simulink model "network_components"  (R2025b)
settings: Solver=VariableStepAuto  StartTime=0.0  StopTime=10.0  RelTol=1e-3
undefined symbols (not defined in the file or in its folder): Bpu, lineParam, Rpu
libraries: ee_lib x8, fl_lib x8, nesl_utility x4, ee_lib_for_power_systems x2
settings Model: Creator=gdudgeon  LastModifiedBy=gdudgeon

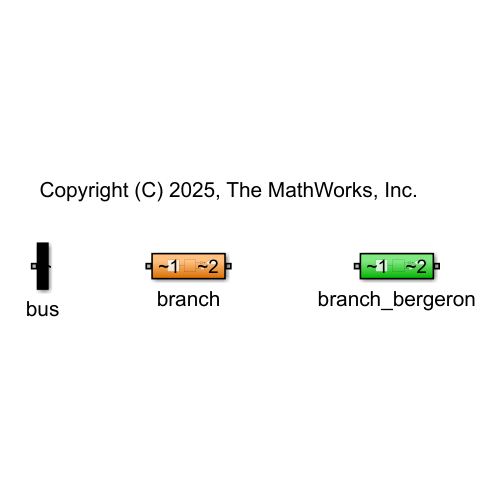
[thumbnail: Simulink's stored preview of the top-level diagram]
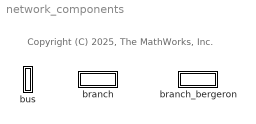
== system network_components ==
  note: Copyright (C) 2025, The MathWorks, Inc.
  branch : Subsystem
  branch_bergeron : Subsystem
  bus : Subsystem

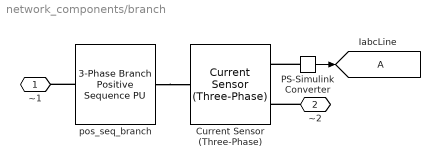
== system network_components/branch ==
  Current Sensor (Three-Phase) : ee_lib/Sensors & Transducers/Current Sensor (Three-Phase)
  IabcLine : Goto  TagVisibility=global
  PS-Simulink Converter : nesl_utility/PS-Simulink Converter  PhysicalDomain=network_engine_domain  SubClassName=ps_output  LeftPortType=input  RightPortType=output  PseudoPeriodic=off  Frequencies=[]  VectorFormat=inherit  Unit=inherit  AffineConversion=off
  pos_seq_branch : ee_lib_for_power_systems/Network Components/3-Phase Branch Positive Sequence PU  Pnom_Fnom=[5e6 60]  Tx=off  Vnom1=5e3  Vnom2=2e3  R=Rpu  X=Xpu  B=Bpu  run_time=on
      settings: SourceProductName=Support Library for Power Systems
  ~1 : PMIOPort  Side=Left
  ~2 : PMIOPort  Port=2  Side=Right
  wires:
  PS-Simulink Converter/1 -> IabcLine/1
  connections:
  PS-Simulink Converter/LConn1 -- Current Sensor (Three-Phase)/RConn1
  ~2/RConn1 -- Current Sensor (Three-Phase)/RConn2
  pos_seq_branch/RConn1 -- Current Sensor (Three-Phase)/LConn1
  pos_seq_branch/LConn1 -- ~1/RConn1

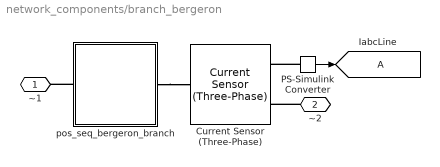
== system network_components/branch_bergeron ==
  Current Sensor (Three-Phase) : ee_lib/Sensors & Transducers/Current Sensor (Three-Phase)
  IabcLine : Goto  TagVisibility=global
  PS-Simulink Converter : nesl_utility/PS-Simulink Converter  PhysicalDomain=network_engine_domain  SubClassName=ps_output  LeftPortType=input  RightPortType=output  PseudoPeriodic=off  Frequencies=[]  VectorFormat=inherit  Unit=inherit  AffineConversion=off
  pos_seq_bergeron_branch : Subsystem  mask{Pnom_Fnom=[5e6 60], Tx=off, Vnom1=5e3, Vnom2=2e3, R=0.1, X=0.01, B=1e-9}
      mask prompts: Pnom_Fnom "Nominal values [Pnom(VA) Fnom(Hz)]"; Tx "Include Ideal Transformer"; Vnom1 "Port 1 Nominal Voltage (Vrms)"; Vnom2 "Nominal Voltage (Vrms)"; R "Series Resistance R (pu)"; X "Series Reactance X (pu)"; B "Shunt Line Charging Susceptance B (pu)"
      mask init:
      | maskObj = Simulink.Mask.get(gcbh);
      | workspaceObj = maskObj.getWorkspace();
      | 
      | Pnom_Vnom = workspaceObj.get('Pnom_Fnom');
      | Vnom1 = workspaceObj.get('Vnom1');
      | Vnom2 = workspaceObj.get('Vnom2');
      | 
      | R = workspaceObj.get('R');
      | X = workspaceObj.get('X');
      | B = workspaceObj.get('B');
      | 
      | R1 = R*Vnom2^2/Pnom_Fnom(1);
      | R0 = R1;
      | 
      | L1 = X*Vnom2^2/Pnom_Fnom(1)/(2*pi*Pnom_Fnom(2));
      | L0 = L1;
      | 
      | C1 = B/(Vnom2^2/Pnom_Fnom(1))/(2*pi*Pnom_Fnom(2));
      | C0 = C1;
      mask Callback Tx:
      | Tx = get_param(gcb,'Tx');
      | 
      | path_Tx  = [gcb,'/Tx'];
      | 
      | mp  ={
      |     'Nominal values [Pnom(VA) Fnom(Hz)]'
      |     'Include Ideal Transformer'
      |     'Port 1 Nominal Voltage (Vrms)'
      |     'Nominal Voltage (Vrms)'
      |     'Series Resistance R (pu)'
      |     'Series Reactance X (pu)'
      |     'Shunt Line Charging Susceptance B (pu)'
      |     };
      | 
      | set_param(gcb,'MaskPrompts',mp)
      | 
      | switch Tx
      | 
      |     case 'off'
      | 
      |         set_param(gcb,'MaskVisibilityString','on,on,off,on,on,on,on')
      |         set_param(path_Tx,'Commented','through')
      | 
      |     case 'on'
      | 
      |         set_param(gcb,'MaskVisibilityString','on,on,on,on,on,on,on')
      |         mp{4} = 'Port 2 Nominal Voltage (Vrms)';
      |         set_param(path_Tx,'Commented','off')
      | 
      | end
      | 
      | set_param(gcb,'MaskPrompts',mp)
      mask DialogControl DescGroupVar Prompt: 3-Phase Branch Positive Sequence PU
      mask DialogControl DescTextVar Prompt: This branch is parameterized from positive sequence data in R, X, B format. Where R is series resistance, X is series reactance and B is line charging susceptance. For series inductance X is positive. For series capacitance, X is negative. When included, the ideal transformer is connected at port 1, and the RLC per-unit values are referred to the voltage at port 2.
      mask DialogControl Container5 Prompt: Parameters
      mask Display: disp('Three-Phase\nBergeron\nPos-Seq (PU)')
  ~1 : PMIOPort  Side=Left
  ~2 : PMIOPort  Port=2  Side=Right
  wires:
  PS-Simulink Converter/1 -> IabcLine/1
  connections:
  pos_seq_bergeron_branch/LConn1 -- ~1/RConn1
  pos_seq_bergeron_branch/RConn1 -- Current Sensor (Three-Phase)/LConn1
  ~2/RConn1 -- Current Sensor (Three-Phase)/RConn2
  PS-Simulink Converter/LConn1 -- Current Sensor (Three-Phase)/RConn1

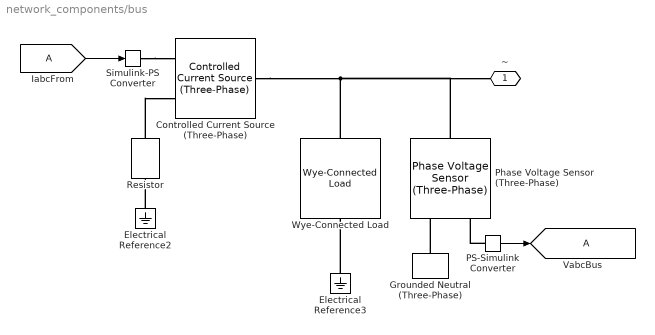
== system network_components/bus ==
  Controlled Current Source (Three-Phase) : ee_lib/Sources/Controlled Current Source (Three-Phase)  input_option=ee.enum.inputType.instantaneous  FRated=60 Hz
      settings: InternalSimscapePortConfiguration="{\"Bottom\":[],\"Left\":[{\"id\":\"S\",\"label\":\"S\",\"type\":\"input\"},{\"id\":\"n\",\"label\":\"n\",\"type\":\"foundation.electrical.electrical\"}],\"Right\":[{\"id\":\"N\",\"label\":\"~\",\"type\":\"foundation.electrical.three_phase\"}],\"Top\":[]}"
  Electrical Reference2 : fl_lib/Electrical/Electrical Elements/Electrical Reference
  Electrical Reference3 : fl_lib/Electrical/Electrical Elements/Electrical Reference
  Grounded Neutral (Three-Phase) : ee_lib/Connectors & References/Grounded Neutral (Three-Phase)
  IabcFrom : From
  PS-Simulink Converter : nesl_utility/PS-Simulink Converter  PhysicalDomain=network_engine_domain  SubClassName=ps_output  LeftPortType=input  RightPortType=output  PseudoPeriodic=off  Frequencies=[]  VectorFormat=inherit  Unit=inherit  AffineConversion=off
  Phase Voltage Sensor (Three-Phase) : ee_lib/Sensors & Transducers/Phase Voltage Sensor (Three-Phase)
  Resistor : fl_lib/Electrical/Electrical Elements/Resistor  R=lineParam.RgI Ohm  i_specify=on  i_priority=High  i=0 A  i_nominal_specify=off  i_nominal_value=1  i_nominal_unit=A  v_specify=on  v_priority=High  v=0 V  v_nominal_specify=off  v_nominal_value=1  v_nominal_unit=V
  Simulink-PS Converter : nesl_utility/Simulink-PS Converter  PhysicalDomain=network_engine_domain  SubClassName=ps_input  LeftPortType=input  RightPortType=output  PseudoPeriodic=off  Frequencies=[]  NoiseDistribution=none  NoiseParameters=[]  Unit=1  AffineConversion=off  FilteringAndDerivatives=zero  SimscapeFilterOrder=1  InputFilterTimeConstant=0.001  UdotUserProvided=0
  VabcBus : Goto  TagVisibility=global
  Wye-Connected Load : ee_lib/Passive/RLC Assemblies/Wye-Connected Load  port_option=ee.enum.threePhasePort.composite  parameterization=ee.enum.rlc.parameterization.ratedpower  component_structure=ee.enum.rlc.structure.R  component_structure_PQ=ee.enum.rlc.structure.ParallelRLC  R=1 Ohm  L=1e-3 H  C=1e-6 F  VRated=24e3 V  FRated=60 Hz  P=1e3 W  Qpos=1e2 A*V  Qneg=-1e2 A*V  R_parasitic=0 Ohm  G_parasitic=0 1/Ohm  R_parasitic_PQ=0 Ohm  G_parasitic_PQ=0 1/Ohm  Vmag0=0 V  Vang0=0 deg  Freq0=60 Hz  IL_specify=off  IL_priority=High  IL=[0, 0, 0] A  IL_nominal_specify=off  IL_nominal_value=1  IL_nominal_unit=A  VC_specify=off  VC_priority=High  VC=[0, 0, 0] V  VC_nominal_specify=off  VC_nominal_value=1  VC_nominal_unit=V
  ~ : PMIOPort  Side=Left
  wires:
  IabcFrom/1 -> Simulink-PS Converter/1
  PS-Simulink Converter/1 -> VabcBus/1
  connections:
  Wye-Connected Load/LConn1 -- Controlled Current Source (Three-Phase)/RConn1 -- Phase Voltage Sensor (Three-Phase)/LConn1 -- ~/RConn1
  Electrical Reference2/LConn1 -- Resistor/LConn1
  Electrical Reference3/LConn1 -- Wye-Connected Load/RConn1
  Simulink-PS Converter/RConn1 -- Controlled Current Source (Three-Phase)/LConn1
  PS-Simulink Converter/LConn1 -- Phase Voltage Sensor (Three-Phase)/RConn1
  Grounded Neutral (Three-Phase)/LConn1 -- Phase Voltage Sensor (Three-Phase)/RConn2
  Resistor/RConn1 -- Controlled Current Source (Three-Phase)/LConn2

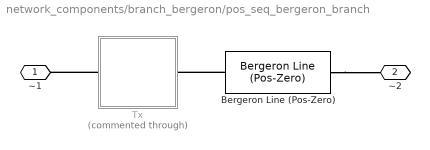
== system network_components/branch_bergeron/pos_seq_bergeron_branch ==
  Bergeron Line (Pos-Zero) : ee_lib_for_power_systems/Network Components/Bergeron Line (Pos-Zero)  length=1  R1_L1_C1=[R1 L1 C1]  R0_L0_C0=[R1 L1 C1]  Ts=5e-5
      settings: SourceProductName=Support Library for Power Systems
  Tx : Subsystem  Commented=through  mask{wr=Vnom1/Vnom2}
      mask prompts: wr "Winding Ratio (V1/V2)"
  ~1 : PMIOPort  Side=Left
  ~2 : PMIOPort  Port=2  Side=Right
  connections:
  Tx/LConn1 -- ~1/RConn1
  Bergeron Line (Pos-Zero)/LConn1 -- Tx/RConn1
  Bergeron Line (Pos-Zero)/RConn1 -- ~2/RConn1

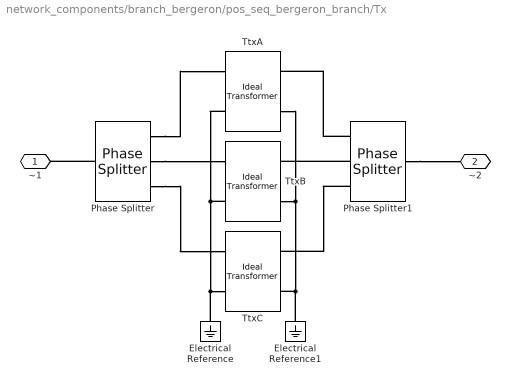
== system network_components/branch_bergeron/pos_seq_bergeron_branch/Tx ==
  Electrical Reference : fl_lib/Electrical/Electrical Elements/Electrical Reference
  Electrical Reference1 : fl_lib/Electrical/Electrical Elements/Electrical Reference
  Phase Splitter : ee_lib/Connectors & References/Phase Splitter
  Phase Splitter1 : ee_lib/Connectors & References/Phase Splitter
  TtxA : fl_lib/Electrical/Electrical Elements/Ideal Transformer  n=wr  i1_specify=on  i1_priority=Low  i1=0 A  i1_nominal_specify=off  i1_nominal_value=1  i1_nominal_unit=A  v1_specify=on  v1_priority=Low  v1=0 V  v1_nominal_specify=off  v1_nominal_value=1  v1_nominal_unit=V  i2_specify=on  i2_priority=Low  i2=0 A  i2_nominal_specify=off  i2_nominal_value=1  i2_nominal_unit=A  v2_specify=on  v2_priority=Low  v2=0 V  v2_nominal_specify=off  v2_nominal_value=1  v2_nominal_unit=V
  TtxB : fl_lib/Electrical/Electrical Elements/Ideal Transformer  n=wr  i1_specify=on  i1_priority=Low  i1=0 A  i1_nominal_specify=off  i1_nominal_value=1  i1_nominal_unit=A  v1_specify=on  v1_priority=Low  v1=0 V  v1_nominal_specify=off  v1_nominal_value=1  v1_nominal_unit=V  i2_specify=on  i2_priority=Low  i2=0 A  i2_nominal_specify=off  i2_nominal_value=1  i2_nominal_unit=A  v2_specify=on  v2_priority=Low  v2=0 V  v2_nominal_specify=off  v2_nominal_value=1  v2_nominal_unit=V
  TtxC : fl_lib/Electrical/Electrical Elements/Ideal Transformer  n=wr  i1_specify=on  i1_priority=Low  i1=0 A  i1_nominal_specify=off  i1_nominal_value=1  i1_nominal_unit=A  v1_specify=on  v1_priority=Low  v1=0 V  v1_nominal_specify=off  v1_nominal_value=1  v1_nominal_unit=V  i2_specify=on  i2_priority=Low  i2=0 A  i2_nominal_specify=off  i2_nominal_value=1  i2_nominal_unit=A  v2_specify=on  v2_priority=Low  v2=0 V  v2_nominal_specify=off  v2_nominal_value=1  v2_nominal_unit=V
  ~1 : PMIOPort  Side=Left
  ~2 : PMIOPort  Port=2  Side=Right
  connections:
  TtxA/LConn2 -- TtxB/LConn2 -- Electrical Reference/LConn1 -- TtxC/LConn2
  Phase Splitter/RConn3 -- TtxC/LConn1
  TtxA/RConn2 -- Electrical Reference1/LConn1 -- TtxC/RConn2 -- TtxB/RConn2
  Phase Splitter1/RConn3 -- TtxC/RConn1
  Phase Splitter1/LConn1 -- ~2/RConn1
  Phase Splitter1/RConn2 -- TtxB/RConn1
  Phase Splitter/RConn2 -- TtxB/LConn1
  Phase Splitter/RConn1 -- TtxA/LConn1
  Phase Splitter1/RConn1 -- TtxA/RConn1
  Phase Splitter/LConn1 -- ~1/RConn1
